simulink model "test_mdl_NI"  (R2018a)
settings: Solver=VariableStepAuto  StartTime=0.0  StopTime=10.0  RelTol=1e-3
(part 3 of 24)

== system test_mdl_NI/To_NI_HIL/MRR ==
  in : Inport
  CAN_DET_AZIMUTH_01[rad] : Subsystem
  CAN_DET_AZIMUTH_02[rad] : Subsystem
  CAN_DET_AZIMUTH_03[rad] : Subsystem
  CAN_DET_ELEVATION_01[rad] : Subsystem
  CAN_DET_ELEVATION_02[rad] : Subsystem
  CAN_DET_ELEVATION_03[rad] : Subsystem
  CAN_DET_RANGE_01[m] : Subsystem
  CAN_DET_RANGE_02[m] : Subsystem
  CAN_DET_RANGE_03[m] : Subsystem
  CAN_DET_RANGE_RATE_01[m|s] : Subsystem
  CAN_DET_RANGE_RATE_02[m|s] : Subsystem
  CAN_DET_RANGE_RATE_03[m|s] : Subsystem
  bus_creator : BusCreator  Inputs=12
  bus_selector : BusSelector  OutputSignals=CAN_DET_RANGE_01[m],CAN_DET_RANGE_RATE_01[m|s],CAN_DET_AZIMUTH_01[rad],CAN_DET_ELEVATION_01[rad],CAN_DET_RANGE_02[m],CAN_DET_RANGE_RATE_02[m|s],CAN_DET_AZIMUTH_02[rad],CAN_DET_ELEVATION_02[rad],CAN_DET_RANGE_03[m],CAN_DET_RANGE_RATE_03[m|s],CAN_DET_AZIMUTH_03[rad],CAN_DET_ELEVATION_03[rad]
  out_port : Outport
  wires:
  bus_creator/1 -> out_port/1  "MRR"
  CAN_DET_RANGE_01[m]/1(out) -> bus_creator/1  "CAN_DET_RANGE_01[m]"
  CAN_DET_RANGE_RATE_01[m|s]/1(out) -> bus_creator/2  "CAN_DET_RANGE_RATE_01[m|s]"
  CAN_DET_AZIMUTH_01[rad]/1(out) -> bus_creator/3  "CAN_DET_AZIMUTH_01[rad]"
  CAN_DET_ELEVATION_01[rad]/1(out) -> bus_creator/4  "CAN_DET_ELEVATION_01[rad]"
  CAN_DET_RANGE_02[m]/1(out) -> bus_creator/5  "CAN_DET_RANGE_02[m]"
  CAN_DET_RANGE_RATE_02[m|s]/1(out) -> bus_creator/6  "CAN_DET_RANGE_RATE_02[m|s]"
  CAN_DET_AZIMUTH_02[rad]/1(out) -> bus_creator/7  "CAN_DET_AZIMUTH_02[rad]"
  CAN_DET_ELEVATION_02[rad]/1(out) -> bus_creator/8  "CAN_DET_ELEVATION_02[rad]"
  CAN_DET_RANGE_03[m]/1(out) -> bus_creator/9  "CAN_DET_RANGE_03[m]"
  CAN_DET_RANGE_RATE_03[m|s]/1(out) -> bus_creator/10  "CAN_DET_RANGE_RATE_03[m|s]"
  CAN_DET_AZIMUTH_03[rad]/1(out) -> bus_creator/11  "CAN_DET_AZIMUTH_03[rad]"
  CAN_DET_ELEVATION_03[rad]/1(out) -> bus_creator/12  "CAN_DET_ELEVATION_03[rad]"
  bus_selector/1 -> CAN_DET_RANGE_01[m]/1(in)  "<CAN_DET_RANGE_01[m]>"
  bus_selector/2 -> CAN_DET_RANGE_RATE_01[m|s]/1(in)  "<CAN_DET_RANGE_RATE_01[m|s]>"
  bus_selector/3 -> CAN_DET_AZIMUTH_01[rad]/1(in)  "<CAN_DET_AZIMUTH_01[rad]>"
  bus_selector/4 -> CAN_DET_ELEVATION_01[rad]/1(in)  "<CAN_DET_ELEVATION_01[rad]>"
  bus_selector/5 -> CAN_DET_RANGE_02[m]/1(in)  "<CAN_DET_RANGE_02[m]>"
  bus_selector/6 -> CAN_DET_RANGE_RATE_02[m|s]/1(in)  "<CAN_DET_RANGE_RATE_02[m|s]>"
  bus_selector/7 -> CAN_DET_AZIMUTH_02[rad]/1(in)  "<CAN_DET_AZIMUTH_02[rad]>"
  bus_selector/8 -> CAN_DET_ELEVATION_02[rad]/1(in)  "<CAN_DET_ELEVATION_02[rad]>"
  bus_selector/9 -> CAN_DET_RANGE_03[m]/1(in)  "<CAN_DET_RANGE_03[m]>"
  bus_selector/10 -> CAN_DET_RANGE_RATE_03[m|s]/1(in)  "<CAN_DET_RANGE_RATE_03[m|s]>"
  bus_selector/11 -> CAN_DET_AZIMUTH_03[rad]/1(in)  "<CAN_DET_AZIMUTH_03[rad]>"
  bus_selector/12 -> CAN_DET_ELEVATION_03[rad]/1(in)  "<CAN_DET_ELEVATION_03[rad]>"
  in/1 -> bus_selector/1

== system test_mdl_NI/To_NI_HIL/SRR_L ==
  in : Inport
  FL_SOD : Subsystem
  RL_SOD : Subsystem
  bus_creator : BusCreator  Inputs=2
  bus_selector : BusSelector  OutputSignals=RL_SOD,FL_SOD
  out_port : Outport
  wires:
  bus_creator/1 -> out_port/1  "SRR_L"
  RL_SOD/1(out_port) -> bus_creator/1  "RL_SOD"
  FL_SOD/1(out_port) -> bus_creator/2  "FL_SOD"
  bus_selector/1 -> RL_SOD/1(in)  "<RL_SOD>"
  bus_selector/2 -> FL_SOD/1(in)  "<FL_SOD>"
  in/1 -> bus_selector/1

== system test_mdl_NI/To_NI_HIL/SRR_R ==
  in : Inport
  FR_SOD : Subsystem
  RR_SOD : Subsystem
  bus_creator : BusCreator  Inputs=2
  bus_selector : BusSelector  OutputSignals=RR_SOD,FR_SOD
  out_port : Outport
  wires:
  bus_creator/1 -> out_port/1  "SRR_R"
  RR_SOD/1(out_port) -> bus_creator/1  "RR_SOD"
  FR_SOD/1(out_port) -> bus_creator/2  "FR_SOD"
  bus_selector/1 -> RR_SOD/1(in)  "<RR_SOD>"
  bus_selector/2 -> FR_SOD/1(in)  "<FR_SOD>"
  in/1 -> bus_selector/1

== system test_mdl_NI/To_NI_HIL/Soft_ABS ==
  in : Inport
  ABS_BrkBst_Data : Subsystem
  Accel_Data : Subsystem
  BrakeSnData_3 : Subsystem
  BrakeSnData_4 : Subsystem
  BrakeSnData_5 : Subsystem
  BrakeSysFeatures : Subsystem
  BrakeSysFeatures_2 : Subsystem
  DesiredTorqBrk : Subsystem
  ToCarSim : Subsystem
  WheelData : Subsystem
  WheelSpeed : Subsystem
  Yaw_Data : Subsystem
  bus_creator : BusCreator  Inputs=12
  bus_selector : BusSelector  OutputSignals=WheelSpeed,WheelData,Accel_Data,Yaw_Data,BrakeSnData_3,DesiredTorqBrk,BrakeSnData_4,BrakeSysFeatures,BrakeSnData_5,ToCarSim,ABS_BrkBst_Data,BrakeSysFeatures_2
  out_port : Outport
  wires:
  bus_creator/1 -> out_port/1  "Soft_ABS"
  WheelSpeed/1(out_port) -> bus_creator/1  "WheelSpeed"
  WheelData/1(out_port) -> bus_creator/2  "WheelData"
  Accel_Data/1(out_port) -> bus_creator/3  "Accel_Data"
  Yaw_Data/1(out_port) -> bus_creator/4  "Yaw_Data"
  BrakeSnData_3/1(out_port) -> bus_creator/5  "BrakeSnData_3"
  DesiredTorqBrk/1(out_port) -> bus_creator/6  "DesiredTorqBrk"
  BrakeSnData_4/1(out_port) -> bus_creator/7  "BrakeSnData_4"
  BrakeSysFeatures/1(out_port) -> bus_creator/8  "BrakeSysFeatures"
  BrakeSnData_5/1(out_port) -> bus_creator/9  "BrakeSnData_5"
  ToCarSim/1(out_port) -> bus_creator/10  "ToCarSim"
  ABS_BrkBst_Data/1(out_port) -> bus_creator/11  "ABS_BrkBst_Data"
  BrakeSysFeatures_2/1(out_port) -> bus_creator/12  "BrakeSysFeatures_2"
  bus_selector/1 -> WheelSpeed/1(in)  "<WheelSpeed>"
  bus_selector/2 -> WheelData/1(in)  "<WheelData>"
  bus_selector/3 -> Accel_Data/1(in)  "<Accel_Data>"
  bus_selector/4 -> Yaw_Data/1(in)  "<Yaw_Data>"
  bus_selector/5 -> BrakeSnData_3/1(in)  "<BrakeSnData_3>"
  bus_selector/6 -> DesiredTorqBrk/1(in)  "<DesiredTorqBrk>"
  bus_selector/7 -> BrakeSnData_4/1(in)  "<BrakeSnData_4>"
  bus_selector/8 -> BrakeSysFeatures/1(in)  "<BrakeSysFeatures>"
  bus_selector/9 -> BrakeSnData_5/1(in)  "<BrakeSnData_5>"
  bus_selector/10 -> ToCarSim/1(in)  "<ToCarSim>"
  bus_selector/11 -> ABS_BrkBst_Data/1(in)  "<ABS_BrkBst_Data>"
  bus_selector/12 -> BrakeSysFeatures_2/1(in)  "<BrakeSysFeatures_2>"
  in/1 -> bus_selector/1

== system test_mdl_NI/To_NI_HIL/Soft_APIM ==
  in : Inport
  out : Outport
  wires:
  in/1 -> out/1

== system test_mdl_NI/To_NI_HIL/Soft_BCM ==
  in : Inport
  BodyInfo_3 : Subsystem
  Cluster_Info1 : Subsystem
  GGCC_Config_Mgmt_ID : Subsystem
  Personality_BCM2_Data : Subsystem
  bus_creator : BusCreator  Inputs=7
  bus_selector : BusSelector  OutputSignals=signal1,Cluster_Info1,BodyInfo_3,GGCC_Config_Mgmt_ID,signal5,signal6,Personality_BCM2_Data
  signal1 : Subsystem
  signal5 : Subsystem
  signal6 : Subsystem
  out_port : Outport
  wires:
  bus_creator/1 -> out_port/1  "Soft_BCM"
  signal1/1(out) -> bus_creator/1  "signal1"
  signal5/1(out) -> bus_creator/5  "signal5"
  signal6/1(out) -> bus_creator/6  "signal6"
  Cluster_Info1/1(out_port) -> bus_creator/2  "Cluster_Info1"
  BodyInfo_3/1(out_port) -> bus_creator/3  "BodyInfo_3"
  GGCC_Config_Mgmt_ID/1(out_port) -> bus_creator/4  "GGCC_Config_Mgmt_ID"
  Personality_BCM2_Data/1(out_port) -> bus_creator/7  "Personality_BCM2_Data"
  bus_selector/1 -> signal1/1(in)  "<signal1>"
  bus_selector/2 -> Cluster_Info1/1(in)  "<Cluster_Info1>"
  bus_selector/3 -> BodyInfo_3/1(in)  "<BodyInfo_3>"
  bus_selector/4 -> GGCC_Config_Mgmt_ID/1(in)  "<GGCC_Config_Mgmt_ID>"
  bus_selector/5 -> signal5/1(in)  "<signal5>"
  bus_selector/6 -> signal6/1(in)  "<signal6>"
  bus_selector/7 -> Personality_BCM2_Data/1(in)  "<Personality_BCM2_Data>"
  in/1 -> bus_selector/1

== system test_mdl_NI/To_NI_HIL/Soft_CCM ==
  in : Inport
  out : Outport
  wires:
  in/1 -> out/1

== system test_mdl_NI/To_NI_HIL/Soft_ECM ==
  in : Inport
  EngBrakeData : Subsystem
  EngVehicleSpThrottle : Subsystem
  EngVehicleSpThrottle2 : Subsystem
  bus_creator : BusCreator  Inputs=3
  bus_selector : BusSelector  OutputSignals=EngVehicleSpThrottle2,EngBrakeData,EngVehicleSpThrottle
  out_port : Outport
  wires:
  bus_creator/1 -> out_port/1  "Soft_ECM"
  EngVehicleSpThrottle2/1(out_port) -> bus_creator/1  "EngVehicleSpThrottle2"
  EngBrakeData/1(out_port) -> bus_creator/2  "EngBrakeData"
  EngVehicleSpThrottle/1(out_port) -> bus_creator/3  "EngVehicleSpThrottle"
  bus_selector/1 -> EngVehicleSpThrottle2/1(in)  "<EngVehicleSpThrottle2>"
  bus_selector/2 -> EngBrakeData/1(in)  "<EngBrakeData>"
  bus_selector/3 -> EngVehicleSpThrottle/1(in)  "<EngVehicleSpThrottle>"
  in/1 -> bus_selector/1

== system test_mdl_NI/To_NI_HIL/Soft_IPC ==
  in : Inport
  out : Outport
  wires:
  in/1 -> out/1

== system test_mdl_NI/To_NI_HIL/Soft_IPMA ==
  in : Inport
  out : Outport
  wires:
  in/1 -> out/1

== system test_mdl_NI/To_NI_HIL/Soft_MRR ==
  in : Inport
  MRR_Detection : Subsystem
  NumOfDetections : Subsystem
  bus_creator : BusCreator  Inputs=2
  bus_selector : BusSelector  OutputSignals=MRR_Detection,NumOfDetections
  out_port : Outport
  wires:
  bus_creator/1 -> out_port/1  "Soft_MRR"
  NumOfDetections/1(out) -> bus_creator/2  "NumOfDetections"
  MRR_Detection/1(out_port) -> bus_creator/1  "MRR_Detection"
  bus_selector/1 -> MRR_Detection/1(in)  "<MRR_Detection>"
  bus_selector/2 -> NumOfDetections/1(in)  "<NumOfDetections>"
  in/1 -> bus_selector/1

== system test_mdl_NI/To_NI_HIL/Soft_PCM ==
  in : Inport
  EngBrakeData : Subsystem
  EngVehicleSpThottle2 : Subsystem
  EngVehicleSpThrottle : Subsystem
  EngineClimateData : Subsystem
  EngineClutchData : Subsystem
  EngineData_7 : Subsystem
  PowertrainData_10 : Subsystem
  TorqueDataEngFlags : Subsystem
  VehicleOperatingModes : Subsystem
  bus_creator : BusCreator  Inputs=9
  bus_selector : BusSelector  OutputSignals=EngBrakeData,EngineClimateData,EngineClutchData,EngVehicleSpThrottle,EngVehicleSpThottle2,VehicleOperatingModes,EngineData_7,TorqueDataEngFlags,PowertrainData_10
  out_port : Outport
  wires:
  bus_creator/1 -> out_port/1  "Soft_PCM"
  EngBrakeData/1(out_port) -> bus_creator/1  "EngBrakeData"
  EngineClimateData/1(out_port) -> bus_creator/2  "EngineClimateData"
  EngineClutchData/1(out_port) -> bus_creator/3  "EngineClutchData"
  EngVehicleSpThrottle/1(out_port) -> bus_creator/4  "EngVehicleSpThrottle"
  EngVehicleSpThottle2/1(out_port) -> bus_creator/5  "EngVehicleSpThottle2"
  VehicleOperatingModes/1(out_port) -> bus_creator/6  "VehicleOperatingModes"
  EngineData_7/1(out_port) -> bus_creator/7  "EngineData_7"
  TorqueDataEngFlags/1(out_port) -> bus_creator/8  "TorqueDataEngFlags"
  PowertrainData_10/1(out_port) -> bus_creator/9  "PowertrainData_10"
  bus_selector/1 -> EngBrakeData/1(in)  "<EngBrakeData>"
  bus_selector/2 -> EngineClimateData/1(in)  "<EngineClimateData>"
  bus_selector/3 -> EngineClutchData/1(in)  "<EngineClutchData>"
  bus_selector/4 -> EngVehicleSpThrottle/1(in)  "<EngVehicleSpThrottle>"
  bus_selector/5 -> EngVehicleSpThottle2/1(in)  "<EngVehicleSpThottle2>"
  bus_selector/6 -> VehicleOperatingModes/1(in)  "<VehicleOperatingModes>"
  bus_selector/7 -> EngineData_7/1(in)  "<EngineData_7>"
  bus_selector/8 -> TorqueDataEngFlags/1(in)  "<TorqueDataEngFlags>"
  bus_selector/9 -> PowertrainData_10/1(in)  "<PowertrainData_10>"
  in/1 -> bus_selector/1

== system test_mdl_NI/To_NI_HIL/Soft_PSCM ==
  in : Inport
  Angle_SteeringWheel : Subsystem
  StePinCompAnEst_D_Qf : Subsystem
  StePinRelInit_An_Sns : Subsystem
  StePw_B_Rq : Subsystem
  SteWhlAngCounter : Subsystem
  WhlAngleCs : Subsystem
  bus_creator : BusCreator  Inputs=6
  bus_selector : BusSelector  OutputSignals=Angle_SteeringWheel,SteWhlAngCounter,WhlAngleCs,StePinRelInit_An_Sns,StePw_B_Rq,StePinCompAnEst_D_Qf
  out_port : Outport
  wires:
  bus_creator/1 -> out_port/1  "Soft_PSCM"
  Angle_SteeringWheel/1(out) -> bus_creator/1  "Angle_SteeringWheel"
  SteWhlAngCounter/1(out) -> bus_creator/2  "SteWhlAngCounter"
  WhlAngleCs/1(out) -> bus_creator/3  "WhlAngleCs"
  StePinRelInit_An_Sns/1(out) -> bus_creator/4  "StePinRelInit_An_Sns"
  StePw_B_Rq/1(out) -> bus_creator/5  "StePw_B_Rq"
  StePinCompAnEst_D_Qf/1(out) -> bus_creator/6  "StePinCompAnEst_D_Qf"
  bus_selector/1 -> Angle_SteeringWheel/1(in)  "<Angle_SteeringWheel>"
  bus_selector/2 -> SteWhlAngCounter/1(in)  "<SteWhlAngCounter>"
  bus_selector/3 -> WhlAngleCs/1(in)  "<WhlAngleCs>"
  bus_selector/4 -> StePinRelInit_An_Sns/1(in)  "<StePinRelInit_An_Sns>"
  bus_selector/5 -> StePw_B_Rq/1(in)  "<StePw_B_Rq>"
  bus_selector/6 -> StePinCompAnEst_D_Qf/1(in)  "<StePinCompAnEst_D_Qf>"
  in/1 -> bus_selector/1

== system test_mdl_NI/To_NI_HIL/Soft_RCM ==
  in : Inport
  Accel_Data : Subsystem
  RCMStatusMessage2 : Subsystem
  Yaw_Data : Subsystem
  bus_creator : BusCreator  Inputs=3
  bus_selector : BusSelector  OutputSignals=Accel_Data,Yaw_Data,RCMStatusMessage2
  out_port : Outport
  wires:
  bus_creator/1 -> out_port/1  "Soft_RCM"
  Accel_Data/1(out_port) -> bus_creator/1  "Accel_Data"
  Yaw_Data/1(out_port) -> bus_creator/2  "Yaw_Data"
  RCMStatusMessage2/1(out_port) -> bus_creator/3  "RCMStatusMessage2"
  bus_selector/1 -> Accel_Data/1(in)  "<Accel_Data>"
  bus_selector/2 -> Yaw_Data/1(in)  "<Yaw_Data>"
  bus_selector/3 -> RCMStatusMessage2/1(in)  "<RCMStatusMessage2>"
  in/1 -> bus_selector/1

== system test_mdl_NI/To_NI_HIL/Soft_SCCM ==
  in : Inport
  Steering_Data : Subsystem
  Steering_Wheel_Data2 : Subsystem
  bus_creator : BusCreator  Inputs=2
  bus_selector : BusSelector  OutputSignals=Steering_Data,Steering_Wheel_Data2
  out_port : Outport
  wires:
  bus_creator/1 -> out_port/1  "Soft_SCCM"
  Steering_Data/1(out_port) -> bus_creator/1  "Steering_Data"
  Steering_Wheel_Data2/1(out_port) -> bus_creator/2  "Steering_Wheel_Data2"
  bus_selector/1 -> Steering_Data/1(in)  "<Steering_Data>"
  bus_selector/2 -> Steering_Wheel_Data2/1(in)  "<Steering_Wheel_Data2>"
  in/1 -> bus_selector/1

== system test_mdl_NI/To_NI_HIL/Soft_TCM ==
  in : Inport
  TransGearData : Subsystem
  bus_creator : BusCreator  Inputs=1
  bus_selector : BusSelector  OutputSignals=TransGearData
  out_port : Outport
  wires:
  bus_creator/1 -> out_port/1  "Soft_TCM"
  TransGearData/1(out_port) -> bus_creator/1  "TransGearData"
  bus_selector/1 -> TransGearData/1(in)  "<TransGearData>"
  in/1 -> bus_selector/1

== system test_mdl_NI/CAN_Signal/ABS_ESC/ABS_AutoSar_NetworkMgt_0x596 ==
  in : Inport
  ABS_AutoSarNMControl : Subsystem
  ABS_AutoSarNMNodeId : Subsystem
  ABS_AutoSarNMReserved1 : Subsystem
  ABS_AutoSarNMReserved2 : Subsystem
  ABS_AutoSarNMReserved3 : Subsystem
  ABS_AutoSarNMReserved4 : Subsystem
  ABS_GWNMProxy : Subsystem
  ABS_GWOnBoardTester : Subsystem
  bus_creator : BusCreator  Inputs=8
  bus_selector : BusSelector  OutputSignals=ABS_AutoSarNMNodeId,ABS_AutoSarNMControl,ABS_AutoSarNMReserved1,ABS_AutoSarNMReserved2,ABS_GWOnBoardTester,ABS_GWNMProxy,ABS_AutoSarNMReserved3,ABS_AutoSarNMReserved4
  out_port : Outport
  wires:
  bus_creator/1 -> out_port/1  "ABS_AutoSar_NetworkMgt_0x596"
  ABS_AutoSarNMNodeId/1(out) -> bus_creator/1  "ABS_AutoSarNMNodeId"
  ABS_AutoSarNMControl/1(out) -> bus_creator/2  "ABS_AutoSarNMControl"
  ABS_AutoSarNMReserved1/1(out) -> bus_creator/3  "ABS_AutoSarNMReserved1"
  ABS_AutoSarNMReserved2/1(out) -> bus_creator/4  "ABS_AutoSarNMReserved2"
  ABS_GWOnBoardTester/1(out) -> bus_creator/5  "ABS_GWOnBoardTester"
  ABS_GWNMProxy/1(out) -> bus_creator/6  "ABS_GWNMProxy"
  ABS_AutoSarNMReserved3/1(out) -> bus_creator/7  "ABS_AutoSarNMReserved3"
  ABS_AutoSarNMReserved4/1(out) -> bus_creator/8  "ABS_AutoSarNMReserved4"
  bus_selector/1 -> ABS_AutoSarNMNodeId/1(in)  "<ABS_AutoSarNMNodeId>"
  bus_selector/2 -> ABS_AutoSarNMControl/1(in)  "<ABS_AutoSarNMControl>"
  bus_selector/3 -> ABS_AutoSarNMReserved1/1(in)  "<ABS_AutoSarNMReserved1>"
  bus_selector/4 -> ABS_AutoSarNMReserved2/1(in)  "<ABS_AutoSarNMReserved2>"
  bus_selector/5 -> ABS_GWOnBoardTester/1(in)  "<ABS_GWOnBoardTester>"
  bus_selector/6 -> ABS_GWNMProxy/1(in)  "<ABS_GWNMProxy>"
  bus_selector/7 -> ABS_AutoSarNMReserved3/1(in)  "<ABS_AutoSarNMReserved3>"
  bus_selector/8 -> ABS_AutoSarNMReserved4/1(in)  "<ABS_AutoSarNMReserved4>"
  in/1 -> bus_selector/1

== system test_mdl_NI/CAN_Signal/ABS_ESC/ABS_BrkBst_Data_0x4B0 ==
  in : Inport
  BrkAutoHold_D_Stat : Subsystem
  BrkBstrVac_P_Actl : Subsystem
  BrkTotTqRqDrv_No_Cnt : Subsystem
  BrkTotTqRqDrv_No_Cs : Subsystem
  BrkTot_Tq_RqDrv : Subsystem
  HsaStat_D_Dsply : Subsystem
  HsaTrnAout_Tq_Rq : Subsystem
  YawStabilityIndex : Subsystem
  bus_creator : BusCreator  Inputs=8
  bus_selector : BusSelector  OutputSignals=BrkBstrVac_P_Actl,YawStabilityIndex,HsaTrnAout_Tq_Rq,BrkTotTqRqDrv_No_Cnt,BrkAutoHold_D_Stat,BrkTot_Tq_RqDrv,HsaStat_D_Dsply,BrkTotTqRqDrv_No_Cs
  out_port : Outport
  wires:
  bus_creator/1 -> out_port/1  "ABS_BrkBst_Data_0x4B0"
  BrkBstrVac_P_Actl/1(out) -> bus_creator/1  "BrkBstrVac_P_Actl"
  YawStabilityIndex/1(out) -> bus_creator/2  "YawStabilityIndex"
  HsaTrnAout_Tq_Rq/1(out) -> bus_creator/3  "HsaTrnAout_Tq_Rq"
  BrkTotTqRqDrv_No_Cnt/1(out) -> bus_creator/4  "BrkTotTqRqDrv_No_Cnt"
  BrkAutoHold_D_Stat/1(out) -> bus_creator/5  "BrkAutoHold_D_Stat"
  BrkTot_Tq_RqDrv/1(out) -> bus_creator/6  "BrkTot_Tq_RqDrv"
  HsaStat_D_Dsply/1(out) -> bus_creator/7  "HsaStat_D_Dsply"
  BrkTotTqRqDrv_No_Cs/1(out) -> bus_creator/8  "BrkTotTqRqDrv_No_Cs"
  bus_selector/1 -> BrkBstrVac_P_Actl/1(in)  "<BrkBstrVac_P_Actl>"
  bus_selector/2 -> YawStabilityIndex/1(in)  "<YawStabilityIndex>"
  bus_selector/3 -> HsaTrnAout_Tq_Rq/1(in)  "<HsaTrnAout_Tq_Rq>"
  bus_selector/4 -> BrkTotTqRqDrv_No_Cnt/1(in)  "<BrkTotTqRqDrv_No_Cnt>"
  bus_selector/5 -> BrkAutoHold_D_Stat/1(in)  "<BrkAutoHold_D_Stat>"
  bus_selector/6 -> BrkTot_Tq_RqDrv/1(in)  "<BrkTot_Tq_RqDrv>"
  bus_selector/7 -> HsaStat_D_Dsply/1(in)  "<HsaStat_D_Dsply>"
  bus_selector/8 -> BrkTotTqRqDrv_No_Cs/1(in)  "<BrkTotTqRqDrv_No_Cs>"
  in/1 -> bus_selector/1

== system test_mdl_NI/CAN_Signal/ABS_ESC/ABS_Rapid_Data_Response_1_0x6B0 ==
  in : Inport
  UUDTABSResponse1 : Subsystem
  bus_creator : BusCreator  Inputs=1
  bus_selector : BusSelector  OutputSignals=UUDTABSResponse1
  out_port : Outport
  wires:
  bus_creator/1 -> out_port/1  "ABS_Rapid_Data_Response_1_0x6B0"
  UUDTABSResponse1/1(out) -> bus_creator/1  "UUDTABSResponse1"
  bus_selector/1 -> UUDTABSResponse1/1(in)  "<UUDTABSResponse1>"
  in/1 -> bus_selector/1

== system test_mdl_NI/CAN_Signal/ABS_ESC/ABS_Rapid_Data_Response_2_0x6B1 ==
  in : Inport
  UUDTABSResponse2 : Subsystem
  bus_creator : BusCreator  Inputs=1
  bus_selector : BusSelector  OutputSignals=UUDTABSResponse2
  out_port : Outport
  wires:
  bus_creator/1 -> out_port/1  "ABS_Rapid_Data_Response_2_0x6B1"
  UUDTABSResponse2/1(out) -> bus_creator/1  "UUDTABSResponse2"
  bus_selector/1 -> UUDTABSResponse2/1(in)  "<UUDTABSResponse2>"
  in/1 -> bus_selector/1

== system test_mdl_NI/CAN_Signal/ABS_ESC/ActiveFronSteering_Req_0x88 ==
  in : Inport
  SteWhlBrkAnRq_No_Cnt : Subsystem
  SteWhlBrkAnRq_No_Cs : Subsystem
  SteWhlBrkOffst_An_Rq : Subsystem
  bus_creator : BusCreator  Inputs=3
  bus_selector : BusSelector  OutputSignals=SteWhlBrkOffst_An_Rq,SteWhlBrkAnRq_No_Cs,SteWhlBrkAnRq_No_Cnt
  out_port : Outport
  wires:
  bus_creator/1 -> out_port/1  "ActiveFronSteering_Req_0x88"
  SteWhlBrkOffst_An_Rq/1(out) -> bus_creator/1  "SteWhlBrkOffst_An_Rq"
  SteWhlBrkAnRq_No_Cs/1(out) -> bus_creator/2  "SteWhlBrkAnRq_No_Cs"
  SteWhlBrkAnRq_No_Cnt/1(out) -> bus_creator/3  "SteWhlBrkAnRq_No_Cnt"
  bus_selector/1 -> SteWhlBrkOffst_An_Rq/1(in)  "<SteWhlBrkOffst_An_Rq>"
  bus_selector/2 -> SteWhlBrkAnRq_No_Cs/1(in)  "<SteWhlBrkAnRq_No_Cs>"
  bus_selector/3 -> SteWhlBrkAnRq_No_Cnt/1(in)  "<SteWhlBrkAnRq_No_Cnt>"
  in/1 -> bus_selector/1

== system test_mdl_NI/CAN_Signal/ABS_ESC/BrakeSnData_3_0x77 ==
  in : Inport
  VehLatComp_A_Actl : Subsystem
  VehLongComp_A_Actl : Subsystem
  VehOverGnd_V_Est : Subsystem
  VehTrvlDir_D_Stat : Subsystem
  VehYawComp_W_Actl : Subsystem
  bus_creator : BusCreator  Inputs=5
  bus_selector : BusSelector  OutputSignals=VehOverGnd_V_Est,VehTrvlDir_D_Stat,VehYawComp_W_Actl,VehLatComp_A_Actl,VehLongComp_A_Actl
  out_port : Outport
  wires:
  bus_creator/1 -> out_port/1  "BrakeSnData_3_0x77"
  VehOverGnd_V_Est/1(out) -> bus_creator/1  "VehOverGnd_V_Est"
  VehTrvlDir_D_Stat/1(out) -> bus_creator/2  "VehTrvlDir_D_Stat"
  VehYawComp_W_Actl/1(out) -> bus_creator/3  "VehYawComp_W_Actl"
  VehLatComp_A_Actl/1(out) -> bus_creator/4  "VehLatComp_A_Actl"
  VehLongComp_A_Actl/1(out) -> bus_creator/5  "VehLongComp_A_Actl"
  bus_selector/1 -> VehOverGnd_V_Est/1(in)  "<VehOverGnd_V_Est>"
  bus_selector/2 -> VehTrvlDir_D_Stat/1(in)  "<VehTrvlDir_D_Stat>"
  bus_selector/3 -> VehYawComp_W_Actl/1(in)  "<VehYawComp_W_Actl>"
  bus_selector/4 -> VehLatComp_A_Actl/1(in)  "<VehLatComp_A_Actl>"
  bus_selector/5 -> VehLongComp_A_Actl/1(in)  "<VehLongComp_A_Actl>"
  in/1 -> bus_selector/1

== system test_mdl_NI/CAN_Signal/ABS_ESC/BrakeSnData_4_0x7D ==
  in : Inport
  BrkTotTqRqArb_No_Cnt : Subsystem
  BrkTotTqRqArb_No_Cs : Subsystem
  BrkTot_Tq_Actl : Subsystem
  BrkTot_Tq_RqArb : Subsystem
  HsaStat_D_Actl : Subsystem
  VehRolComp_W_Actl : Subsystem
  VehVertComp_A_Actl : Subsystem
  bus_creator : BusCreator  Inputs=7
  bus_selector : BusSelector  OutputSignals=HsaStat_D_Actl,BrkTot_Tq_RqArb,BrkTotTqRqArb_No_Cs,BrkTotTqRqArb_No_Cnt,BrkTot_Tq_Actl,VehVertComp_A_Actl,VehRolComp_W_Actl
  out_port : Outport
  wires:
  bus_creator/1 -> out_port/1  "BrakeSnData_4_0x7D"
  HsaStat_D_Actl/1(out) -> bus_creator/1  "HsaStat_D_Actl"
  BrkTot_Tq_RqArb/1(out) -> bus_creator/2  "BrkTot_Tq_RqArb"
  BrkTotTqRqArb_No_Cs/1(out) -> bus_creator/3  "BrkTotTqRqArb_No_Cs"
  BrkTotTqRqArb_No_Cnt/1(out) -> bus_creator/4  "BrkTotTqRqArb_No_Cnt"
  BrkTot_Tq_Actl/1(out) -> bus_creator/5  "BrkTot_Tq_Actl"
  VehVertComp_A_Actl/1(out) -> bus_creator/6  "VehVertComp_A_Actl"
  VehRolComp_W_Actl/1(out) -> bus_creator/7  "VehRolComp_W_Actl"
  bus_selector/1 -> HsaStat_D_Actl/1(in)  "<HsaStat_D_Actl>"
  bus_selector/2 -> BrkTot_Tq_RqArb/1(in)  "<BrkTot_Tq_RqArb>"
  bus_selector/3 -> BrkTotTqRqArb_No_Cs/1(in)  "<BrkTotTqRqArb_No_Cs>"
  bus_selector/4 -> BrkTotTqRqArb_No_Cnt/1(in)  "<BrkTotTqRqArb_No_Cnt>"
  bus_selector/5 -> BrkTot_Tq_Actl/1(in)  "<BrkTot_Tq_Actl>"
  bus_selector/6 -> VehVertComp_A_Actl/1(in)  "<VehVertComp_A_Actl>"
  bus_selector/7 -> VehRolComp_W_Actl/1(in)  "<VehRolComp_W_Actl>"
  in/1 -> bus_selector/1

== system test_mdl_NI/CAN_Signal/ABS_ESC/BrakeSnData_5_0x76 ==
  in : Inport
  AwdLck_Tq_RqMn : Subsystem
  AwdLck_Tq_RqMx : Subsystem
  BrkCtrFnd_B_Stat : Subsystem
  DrvSte_D_Stat : Subsystem
  DrvSte_Tq_Rq : Subsystem
  EmgcyBrkLamp_D_Rq : Subsystem
  SteWhlCompAnEst_D_Qf : Subsystem
  SteWhlComp_An_Est : Subsystem
  StopLamp_B_RqBrk : Subsystem
  bus_creator : BusCreator  Inputs=9
  bus_selector : BusSelector  OutputSignals=StopLamp_B_RqBrk,SteWhlComp_An_Est,SteWhlCompAnEst_D_Qf,EmgcyBrkLamp_D_Rq,DrvSte_D_Stat,DrvSte_Tq_Rq,BrkCtrFnd_B_Stat,AwdLck_Tq_RqMx,AwdLck_Tq_RqMn
  out_port : Outport
  wires:
  bus_creator/1 -> out_port/1  "BrakeSnData_5_0x76"
  StopLamp_B_RqBrk/1(out) -> bus_creator/1  "StopLamp_B_RqBrk"
  SteWhlComp_An_Est/1(out) -> bus_creator/2  "SteWhlComp_An_Est"
  SteWhlCompAnEst_D_Qf/1(out) -> bus_creator/3  "SteWhlCompAnEst_D_Qf"
  EmgcyBrkLamp_D_Rq/1(out) -> bus_creator/4  "EmgcyBrkLamp_D_Rq"
  DrvSte_D_Stat/1(out) -> bus_creator/5  "DrvSte_D_Stat"
  DrvSte_Tq_Rq/1(out) -> bus_creator/6  "DrvSte_Tq_Rq"
  BrkCtrFnd_B_Stat/1(out) -> bus_creator/7  "BrkCtrFnd_B_Stat"
  AwdLck_Tq_RqMx/1(out) -> bus_creator/8  "AwdLck_Tq_RqMx"
  AwdLck_Tq_RqMn/1(out) -> bus_creator/9  "AwdLck_Tq_RqMn"
  bus_selector/1 -> StopLamp_B_RqBrk/1(in)  "<StopLamp_B_RqBrk>"
  bus_selector/2 -> SteWhlComp_An_Est/1(in)  "<SteWhlComp_An_Est>"
  bus_selector/3 -> SteWhlCompAnEst_D_Qf/1(in)  "<SteWhlCompAnEst_D_Qf>"
  bus_selector/4 -> EmgcyBrkLamp_D_Rq/1(in)  "<EmgcyBrkLamp_D_Rq>"
  bus_selector/5 -> DrvSte_D_Stat/1(in)  "<DrvSte_D_Stat>"
  bus_selector/6 -> DrvSte_Tq_Rq/1(in)  "<DrvSte_Tq_Rq>"
  bus_selector/7 -> BrkCtrFnd_B_Stat/1(in)  "<BrkCtrFnd_B_Stat>"
  bus_selector/8 -> AwdLck_Tq_RqMx/1(in)  "<AwdLck_Tq_RqMx>"
  bus_selector/9 -> AwdLck_Tq_RqMn/1(in)  "<AwdLck_Tq_RqMn>"
  in/1 -> bus_selector/1

== system test_mdl_NI/CAN_Signal/ABS_ESC/BrakeSnData_6_0x414 ==
  in : Inport
  StePinOffst_An_Est : Subsystem
  StePinOffst_D_Stat : Subsystem
  StePinOffst_No_Cnt : Subsystem
  StePinOffst_No_Cs : Subsystem
  bus_creator : BusCreator  Inputs=4
  bus_selector : BusSelector  OutputSignals=StePinOffst_An_Est,StePinOffst_D_Stat,StePinOffst_No_Cnt,StePinOffst_No_Cs
  out_port : Outport
  wires:
  bus_creator/1 -> out_port/1  "BrakeSnData_6_0x414"
  StePinOffst_An_Est/1(out) -> bus_creator/1  "StePinOffst_An_Est"
  StePinOffst_D_Stat/1(out) -> bus_creator/2  "StePinOffst_D_Stat"
  StePinOffst_No_Cnt/1(out) -> bus_creator/3  "StePinOffst_No_Cnt"
  StePinOffst_No_Cs/1(out) -> bus_creator/4  "StePinOffst_No_Cs"
  bus_selector/1 -> StePinOffst_An_Est/1(in)  "<StePinOffst_An_Est>"
  bus_selector/2 -> StePinOffst_D_Stat/1(in)  "<StePinOffst_D_Stat>"
  bus_selector/3 -> StePinOffst_No_Cnt/1(in)  "<StePinOffst_No_Cnt>"
  bus_selector/4 -> StePinOffst_No_Cs/1(in)  "<StePinOffst_No_Cs>"
  in/1 -> bus_selector/1

== system test_mdl_NI/CAN_Signal/ABS_ESC/BrakeSysFeatures_0x415 ==
  in : Inport
  BrkFluidLvl_D_Stat : Subsystem
  LsmcBrkDecel_D_Stat : Subsystem
  VehStab_D_Stat : Subsystem
  VehVActlBrk_D_Qf : Subsystem
  VehVActlBrk_No_Cnt : Subsystem
  VehVActlBrk_No_Cs : Subsystem
  VehYawLin_W_Rq : Subsystem
  VehYawNonLin_W_Rq : Subsystem
  Veh_V_ActlBrk : Subsystem
  bus_creator : BusCreator  Inputs=9
  bus_selector : BusSelector  OutputSignals=Veh_V_ActlBrk,VehVActlBrk_D_Qf,VehVActlBrk_No_Cnt,BrkFluidLvl_D_Stat,VehVActlBrk_No_Cs,LsmcBrkDecel_D_Stat,VehYawLin_W_Rq,VehStab_D_Stat,VehYawNonLin_W_Rq
  out_port : Outport
  wires:
  bus_creator/1 -> out_port/1  "BrakeSysFeatures_0x415"
  Veh_V_ActlBrk/1(out) -> bus_creator/1  "Veh_V_ActlBrk"
  VehVActlBrk_D_Qf/1(out) -> bus_creator/2  "VehVActlBrk_D_Qf"
  VehVActlBrk_No_Cnt/1(out) -> bus_creator/3  "VehVActlBrk_No_Cnt"
  BrkFluidLvl_D_Stat/1(out) -> bus_creator/4  "BrkFluidLvl_D_Stat"
  VehVActlBrk_No_Cs/1(out) -> bus_creator/5  "VehVActlBrk_No_Cs"
  LsmcBrkDecel_D_Stat/1(out) -> bus_creator/6  "LsmcBrkDecel_D_Stat"
  VehYawLin_W_Rq/1(out) -> bus_creator/7  "VehYawLin_W_Rq"
  VehStab_D_Stat/1(out) -> bus_creator/8  "VehStab_D_Stat"
  VehYawNonLin_W_Rq/1(out) -> bus_creator/9  "VehYawNonLin_W_Rq"
  bus_selector/1 -> Veh_V_ActlBrk/1(in)  "<Veh_V_ActlBrk>"
  bus_selector/2 -> VehVActlBrk_D_Qf/1(in)  "<VehVActlBrk_D_Qf>"
  bus_selector/3 -> VehVActlBrk_No_Cnt/1(in)  "<VehVActlBrk_No_Cnt>"
  bus_selector/4 -> BrkFluidLvl_D_Stat/1(in)  "<BrkFluidLvl_D_Stat>"
  bus_selector/5 -> VehVActlBrk_No_Cs/1(in)  "<VehVActlBrk_No_Cs>"
  bus_selector/6 -> LsmcBrkDecel_D_Stat/1(in)  "<LsmcBrkDecel_D_Stat>"
  bus_selector/7 -> VehYawLin_W_Rq/1(in)  "<VehYawLin_W_Rq>"
  bus_selector/8 -> VehStab_D_Stat/1(in)  "<VehStab_D_Stat>"
  bus_selector/9 -> VehYawNonLin_W_Rq/1(in)  "<VehYawNonLin_W_Rq>"
  in/1 -> bus_selector/1

== system test_mdl_NI/CAN_Signal/ABS_ESC/BrakeSysFeatures_2_0x416 ==
  in : Inport
  Abs_B_Falt : Subsystem
  BpedMove_D_Actl : Subsystem
  BpedMove_No_Cnt : Subsystem
  BrkBstrVac_B_Rq : Subsystem
  BrkLamp_B_Rq : Subsystem
  ChimeBrk_B_Rq : Subsystem
  DrvAntiLckLamp_D_Rq : Subsystem
  DrvHdcLampInfo_D_Rq : Subsystem
  DrvHdcMsg_D_Rq : Subsystem
  DrvHdcWarnInfo_D_Rq : Subsystem
  DrvSlipCtlLamp_D_Rq : Subsystem
  DrvSlipCtlMde_D_Ind : Subsystem
  HILL_DESC_MC : Subsystem
  HdcMde_D_Actl : Subsystem
  HsaMde_D_Mem : Subsystem
  RearDiffElckrOpen_B_Rq : Subsystem
  RearDiffLck_Tq2_RqMx : Subsystem
  StabCtlBrk_B_Avail : Subsystem
  TCMode : Subsystem
  TRLR_SWAY_CONFIG_STAT : Subsystem
  TRLR_SWAY_EVNT_IN_PROG : Subsystem
  bus_creator : BusCreator  Inputs=21
  bus_selector : BusSelector  OutputSignals=BpedMove_D_Actl,Abs_B_Falt,StabCtlBrk_B_Avail,BpedMove_No_Cnt,TCMode,ChimeBrk_B_Rq,BrkLamp_B_Rq,DrvHdcLampInfo_D_Rq,DrvHdcMsg_D_Rq,HdcMde_D_Actl,BrkBstrVac_B_Rq,TRLR_SWAY_CONFIG_STAT,TRLR_SWAY_EVNT_IN_PROG,DrvHdcWarnInfo_D_Rq,HsaMde_D_Mem,HILL_DESC_MC,DrvSlipCtlMde_D_Ind,DrvSlipCtlLamp_D_Rq,RearDiffElckrOpen_B_Rq,DrvAntiLckLamp_D_Rq,RearDiffLck_Tq2_RqMx
  out_port : Outport
  wires:
  bus_creator/1 -> out_port/1  "BrakeSysFeatures_2_0x416"
  BpedMove_D_Actl/1(out) -> bus_creator/1  "BpedMove_D_Actl"
  Abs_B_Falt/1(out) -> bus_creator/2  "Abs_B_Falt"
  StabCtlBrk_B_Avail/1(out) -> bus_creator/3  "StabCtlBrk_B_Avail"
  BpedMove_No_Cnt/1(out) -> bus_creator/4  "BpedMove_No_Cnt"
  TCMode/1(out) -> bus_creator/5  "TCMode"
  ChimeBrk_B_Rq/1(out) -> bus_creator/6  "ChimeBrk_B_Rq"
  BrkLamp_B_Rq/1(out) -> bus_creator/7  "BrkLamp_B_Rq"
  DrvHdcLampInfo_D_Rq/1(out) -> bus_creator/8  "DrvHdcLampInfo_D_Rq"
  DrvHdcMsg_D_Rq/1(out) -> bus_creator/9  "DrvHdcMsg_D_Rq"
  HdcMde_D_Actl/1(out) -> bus_creator/10  "HdcMde_D_Actl"
  BrkBstrVac_B_Rq/1(out) -> bus_creator/11  "BrkBstrVac_B_Rq"
  TRLR_SWAY_CONFIG_STAT/1(out) -> bus_creator/12  "TRLR_SWAY_CONFIG_STAT"
  TRLR_SWAY_EVNT_IN_PROG/1(out) -> bus_creator/13  "TRLR_SWAY_EVNT_IN_PROG"
  DrvHdcWarnInfo_D_Rq/1(out) -> bus_creator/14  "DrvHdcWarnInfo_D_Rq"
  HsaMde_D_Mem/1(out) -> bus_creator/15  "HsaMde_D_Mem"
  HILL_DESC_MC/1(out) -> bus_creator/16  "HILL_DESC_MC"
  DrvSlipCtlMde_D_Ind/1(out) -> bus_creator/17  "DrvSlipCtlMde_D_Ind"
  DrvSlipCtlLamp_D_Rq/1(out) -> bus_creator/18  "DrvSlipCtlLamp_D_Rq"
  RearDiffElckrOpen_B_Rq/1(out) -> bus_creator/19  "RearDiffElckrOpen_B_Rq"
  DrvAntiLckLamp_D_Rq/1(out) -> bus_creator/20  "DrvAntiLckLamp_D_Rq"
  RearDiffLck_Tq2_RqMx/1(out) -> bus_creator/21  "RearDiffLck_Tq2_RqMx"
  bus_selector/1 -> BpedMove_D_Actl/1(in)  "<BpedMove_D_Actl>"
  bus_selector/2 -> Abs_B_Falt/1(in)  "<Abs_B_Falt>"
  bus_selector/3 -> StabCtlBrk_B_Avail/1(in)  "<StabCtlBrk_B_Avail>"
  bus_selector/4 -> BpedMove_No_Cnt/1(in)  "<BpedMove_No_Cnt>"
  bus_selector/5 -> TCMode/1(in)  "<TCMode>"
  bus_selector/6 -> ChimeBrk_B_Rq/1(in)  "<ChimeBrk_B_Rq>"
  bus_selector/7 -> BrkLamp_B_Rq/1(in)  "<BrkLamp_B_Rq>"
  bus_selector/8 -> DrvHdcLampInfo_D_Rq/1(in)  "<DrvHdcLampInfo_D_Rq>"
  bus_selector/9 -> DrvHdcMsg_D_Rq/1(in)  "<DrvHdcMsg_D_Rq>"
  bus_selector/10 -> HdcMde_D_Actl/1(in)  "<HdcMde_D_Actl>"
  bus_selector/11 -> BrkBstrVac_B_Rq/1(in)  "<BrkBstrVac_B_Rq>"
  bus_selector/12 -> TRLR_SWAY_CONFIG_STAT/1(in)  "<TRLR_SWAY_CONFIG_STAT>"
  bus_selector/13 -> TRLR_SWAY_EVNT_IN_PROG/1(in)  "<TRLR_SWAY_EVNT_IN_PROG>"
  bus_selector/14 -> DrvHdcWarnInfo_D_Rq/1(in)  "<DrvHdcWarnInfo_D_Rq>"
  bus_selector/15 -> HsaMde_D_Mem/1(in)  "<HsaMde_D_Mem>"
  bus_selector/16 -> HILL_DESC_MC/1(in)  "<HILL_DESC_MC>"
  bus_selector/17 -> DrvSlipCtlMde_D_Ind/1(in)  "<DrvSlipCtlMde_D_Ind>"
  bus_selector/18 -> DrvSlipCtlLamp_D_Rq/1(in)  "<DrvSlipCtlLamp_D_Rq>"
  bus_selector/19 -> RearDiffElckrOpen_B_Rq/1(in)  "<RearDiffElckrOpen_B_Rq>"
  bus_selector/20 -> DrvAntiLckLamp_D_Rq/1(in)  "<DrvAntiLckLamp_D_Rq>"
  bus_selector/21 -> RearDiffLck_Tq2_RqMx/1(in)  "<RearDiffLck_Tq2_RqMx>"
  in/1 -> bus_selector/1

== system test_mdl_NI/CAN_Signal/ABS_ESC/BrakeSysFeatures_3_0x41E ==
  in : Inport
  ApaBrk_D_Stat : Subsystem
  AutoHoldMde_D_Ind : Subsystem
  AutoHoldMsgTxt_D_Rq : Subsystem
  AutoHoldSwMde_B_Ind : Subsystem
  BrkBstrVac_D_Stat : Subsystem
  BrkMdeInhbt_B_RqDsply : Subsystem
  CtaBrk_D_Stat : Subsystem
  DrvSlipCtlMdeMsg_D_Rq : Subsystem
  DrvSlipCtlOffLamp_D_Rq : Subsystem
  RbaBrk_D_Stat : Subsystem
  SelDrvMdeAwd_D_Rq : Subsystem
  SelDrvMdeChassis2_D_Rq : Subsystem
  SelDrvMdeChassis_D_Rq : Subsystem
  TrailCtlMsgTxt_D_Rq : Subsystem
  TrailCtl_D_Stat : Subsystem
  bus_creator : BusCreator  Inputs=15
  bus_selector : BusSelector  OutputSignals=AutoHoldMsgTxt_D_Rq,AutoHoldSwMde_B_Ind,AutoHoldMde_D_Ind,DrvSlipCtlMdeMsg_D_Rq,BrkMdeInhbt_B_RqDsply,DrvSlipCtlOffLamp_D_Rq,BrkBstrVac_D_Stat,SelDrvMdeAwd_D_Rq,SelDrvMdeChassis_D_Rq,ApaBrk_D_Stat,CtaBrk_D_Stat,SelDrvMdeChassis2_D_Rq,TrailCtl_D_Stat,TrailCtlMsgTxt_D_Rq,RbaBrk_D_Stat
  out_port : Outport
  wires:
  bus_creator/1 -> out_port/1  "BrakeSysFeatures_3_0x41E"
  AutoHoldMsgTxt_D_Rq/1(out) -> bus_creator/1  "AutoHoldMsgTxt_D_Rq"
  AutoHoldSwMde_B_Ind/1(out) -> bus_creator/2  "AutoHoldSwMde_B_Ind"
  AutoHoldMde_D_Ind/1(out) -> bus_creator/3  "AutoHoldMde_D_Ind"
  DrvSlipCtlMdeMsg_D_Rq/1(out) -> bus_creator/4  "DrvSlipCtlMdeMsg_D_Rq"
  BrkMdeInhbt_B_RqDsply/1(out) -> bus_creator/5  "BrkMdeInhbt_B_RqDsply"
  DrvSlipCtlOffLamp_D_Rq/1(out) -> bus_creator/6  "DrvSlipCtlOffLamp_D_Rq"
  BrkBstrVac_D_Stat/1(out) -> bus_creator/7  "BrkBstrVac_D_Stat"
  SelDrvMdeAwd_D_Rq/1(out) -> bus_creator/8  "SelDrvMdeAwd_D_Rq"
  SelDrvMdeChassis_D_Rq/1(out) -> bus_creator/9  "SelDrvMdeChassis_D_Rq"
  ApaBrk_D_Stat/1(out) -> bus_creator/10  "ApaBrk_D_Stat"
  CtaBrk_D_Stat/1(out) -> bus_creator/11  "CtaBrk_D_Stat"
  SelDrvMdeChassis2_D_Rq/1(out) -> bus_creator/12  "SelDrvMdeChassis2_D_Rq"
  TrailCtl_D_Stat/1(out) -> bus_creator/13  "TrailCtl_D_Stat"
  TrailCtlMsgTxt_D_Rq/1(out) -> bus_creator/14  "TrailCtlMsgTxt_D_Rq"
  RbaBrk_D_Stat/1(out) -> bus_creator/15  "RbaBrk_D_Stat"
  bus_selector/1 -> AutoHoldMsgTxt_D_Rq/1(in)  "<AutoHoldMsgTxt_D_Rq>"
  bus_selector/2 -> AutoHoldSwMde_B_Ind/1(in)  "<AutoHoldSwMde_B_Ind>"
  bus_selector/3 -> AutoHoldMde_D_Ind/1(in)  "<AutoHoldMde_D_Ind>"
  bus_selector/4 -> DrvSlipCtlMdeMsg_D_Rq/1(in)  "<DrvSlipCtlMdeMsg_D_Rq>"
  bus_selector/5 -> BrkMdeInhbt_B_RqDsply/1(in)  "<BrkMdeInhbt_B_RqDsply>"
  bus_selector/6 -> DrvSlipCtlOffLamp_D_Rq/1(in)  "<DrvSlipCtlOffLamp_D_Rq>"
  bus_selector/7 -> BrkBstrVac_D_Stat/1(in)  "<BrkBstrVac_D_Stat>"
  bus_selector/8 -> SelDrvMdeAwd_D_Rq/1(in)  "<SelDrvMdeAwd_D_Rq>"
  bus_selector/9 -> SelDrvMdeChassis_D_Rq/1(in)  "<SelDrvMdeChassis_D_Rq>"
  bus_selector/10 -> ApaBrk_D_Stat/1(in)  "<ApaBrk_D_Stat>"
  bus_selector/11 -> CtaBrk_D_Stat/1(in)  "<CtaBrk_D_Stat>"
  bus_selector/12 -> SelDrvMdeChassis2_D_Rq/1(in)  "<SelDrvMdeChassis2_D_Rq>"
  bus_selector/13 -> TrailCtl_D_Stat/1(in)  "<TrailCtl_D_Stat>"
  bus_selector/14 -> TrailCtlMsgTxt_D_Rq/1(in)  "<TrailCtlMsgTxt_D_Rq>"
  bus_selector/15 -> RbaBrk_D_Stat/1(in)  "<RbaBrk_D_Stat>"
  in/1 -> bus_selector/1

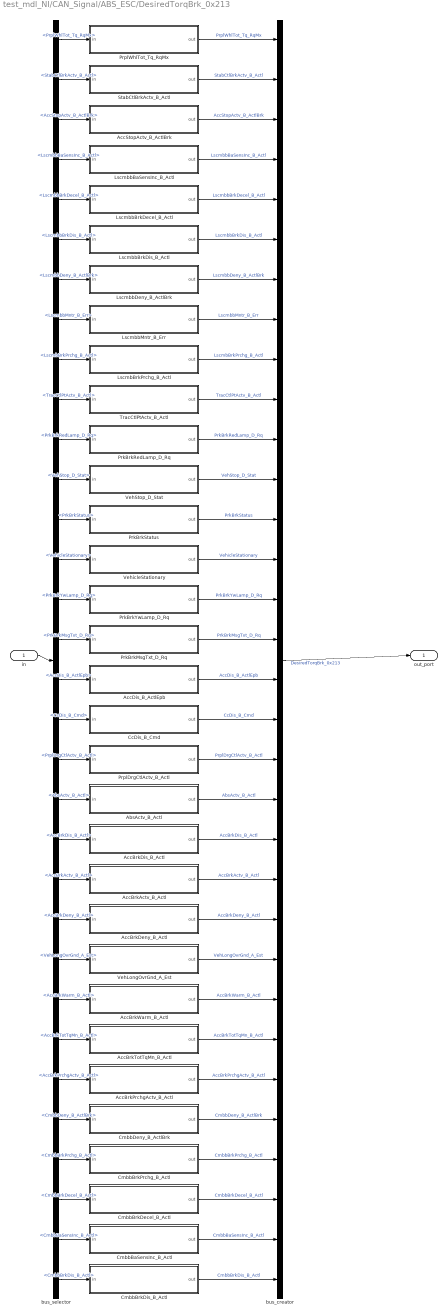
== system test_mdl_NI/CAN_Signal/ABS_ESC/DesiredTorqBrk_0x213 ==
  in : Inport
  AbsActv_B_Actl : Subsystem
  AccBrkActv_B_Actl : Subsystem
  AccBrkDeny_B_Actl : Subsystem
  AccBrkDis_B_Actl : Subsystem
  AccBrkPrchgActv_B_Actl : Subsystem
  AccBrkTotTqMn_B_Actl : Subsystem
  AccBrkWarm_B_Actl : Subsystem
  AccDis_B_ActlEpb : Subsystem
  AccStopActv_B_ActlBrk : Subsystem
  CcDis_B_Cmd : Subsystem
  CmbbBaSensInc_B_Actl : Subsystem
  CmbbBrkDecel_B_Actl : Subsystem
  CmbbBrkDis_B_Actl : Subsystem
  CmbbBrkPrchg_B_Actl : Subsystem
  CmbbDeny_B_ActlBrk : Subsystem
  LscmbBrkPrchg_B_Actl : Subsystem
  LscmbbBaSensInc_B_Actl : Subsystem
  LscmbbBrkDecel_B_Actl : Subsystem
  LscmbbBrkDis_B_Actl : Subsystem
  LscmbbDeny_B_ActlBrk : Subsystem
  LscmbbMntr_B_Err : Subsystem
  PrkBrkMsgTxt_D_Rq : Subsystem
  PrkBrkRedLamp_D_Rq : Subsystem
  PrkBrkStatus : Subsystem
  PrkBrkYwLamp_D_Rq : Subsystem
  PrplDrgCtlActv_B_Actl : Subsystem
  PrplWhlTot_Tq_RqMx : Subsystem
  StabCtlBrkActv_B_Actl : Subsystem
  TracCtlPtActv_B_Actl : Subsystem
  VehLongOvrGnd_A_Est : Subsystem
  VehStop_D_Stat : Subsystem
  VehicleStationary : Subsystem
  bus_creator : BusCreator  Inputs=32
  bus_selector : BusSelector  OutputSignals=PrplWhlTot_Tq_RqMx,StabCtlBrkActv_B_Actl,AccStopActv_B_ActlBrk,LscmbbBaSensInc_B_Actl,LscmbbBrkDecel_B_Actl,LscmbbBrkDis_B_Actl,LscmbbDeny_B_ActlBrk,LscmbbMntr_B_Err,LscmbBrkPrchg_B_Actl,TracCtlPtActv_B_Actl,PrkBrkRedLamp_D_Rq,VehStop_D_Stat,PrkBrkStatus,VehicleStationary,PrkBrkYwLamp_D_Rq,PrkBrkMsgTxt_D_Rq,AccDis_B_ActlEpb,CcDis_B_Cmd,PrplDrgCtlActv_B_Actl,AbsActv_B_Actl,AccBrkDis_B_Actl,AccBrkActv_B_Actl,AccBrkDeny_B_Actl,VehLongOvrGnd_A_Est,AccBrkWarm_B_Actl,AccBrkTotTqMn_B_Actl,AccBrkPrchgActv_B_Actl,CmbbDeny_B_ActlBrk,CmbbBrkPrchg_B_Actl,CmbbBrkDecel_B_Actl,CmbbBaSensInc_B_Actl,CmbbBrkDis_B_Actl
  out_port : Outport
  wires:
  bus_creator/1 -> out_port/1  "DesiredTorqBrk_0x213"
  PrplWhlTot_Tq_RqMx/1(out) -> bus_creator/1  "PrplWhlTot_Tq_RqMx"
  StabCtlBrkActv_B_Actl/1(out) -> bus_creator/2  "StabCtlBrkActv_B_Actl"
  AccStopActv_B_ActlBrk/1(out) -> bus_creator/3  "AccStopActv_B_ActlBrk"
  LscmbbBaSensInc_B_Actl/1(out) -> bus_creator/4  "LscmbbBaSensInc_B_Actl"
  LscmbbBrkDecel_B_Actl/1(out) -> bus_creator/5  "LscmbbBrkDecel_B_Actl"
  LscmbbBrkDis_B_Actl/1(out) -> bus_creator/6  "LscmbbBrkDis_B_Actl"
  LscmbbDeny_B_ActlBrk/1(out) -> bus_creator/7  "LscmbbDeny_B_ActlBrk"
  LscmbbMntr_B_Err/1(out) -> bus_creator/8  "LscmbbMntr_B_Err"
  LscmbBrkPrchg_B_Actl/1(out) -> bus_creator/9  "LscmbBrkPrchg_B_Actl"
  TracCtlPtActv_B_Actl/1(out) -> bus_creator/10  "TracCtlPtActv_B_Actl"
  PrkBrkRedLamp_D_Rq/1(out) -> bus_creator/11  "PrkBrkRedLamp_D_Rq"
  VehStop_D_Stat/1(out) -> bus_creator/12  "VehStop_D_Stat"
  PrkBrkStatus/1(out) -> bus_creator/13  "PrkBrkStatus"
  VehicleStationary/1(out) -> bus_creator/14  "VehicleStationary"
  PrkBrkYwLamp_D_Rq/1(out) -> bus_creator/15  "PrkBrkYwLamp_D_Rq"
  PrkBrkMsgTxt_D_Rq/1(out) -> bus_creator/16  "PrkBrkMsgTxt_D_Rq"
  AccDis_B_ActlEpb/1(out) -> bus_creator/17  "AccDis_B_ActlEpb"
  CcDis_B_Cmd/1(out) -> bus_creator/18  "CcDis_B_Cmd"
  PrplDrgCtlActv_B_Actl/1(out) -> bus_creator/19  "PrplDrgCtlActv_B_Actl"
  AbsActv_B_Actl/1(out) -> bus_creator/20  "AbsActv_B_Actl"
  AccBrkDis_B_Actl/1(out) -> bus_creator/21  "AccBrkDis_B_Actl"
  AccBrkActv_B_Actl/1(out) -> bus_creator/22  "AccBrkActv_B_Actl"
  AccBrkDeny_B_Actl/1(out) -> bus_creator/23  "AccBrkDeny_B_Actl"
  VehLongOvrGnd_A_Est/1(out) -> bus_creator/24  "VehLongOvrGnd_A_Est"
  AccBrkWarm_B_Actl/1(out) -> bus_creator/25  "AccBrkWarm_B_Actl"
  AccBrkTotTqMn_B_Actl/1(out) -> bus_creator/26  "AccBrkTotTqMn_B_Actl"
  AccBrkPrchgActv_B_Actl/1(out) -> bus_creator/27  "AccBrkPrchgActv_B_Actl"
  CmbbDeny_B_ActlBrk/1(out) -> bus_creator/28  "CmbbDeny_B_ActlBrk"
  CmbbBrkPrchg_B_Actl/1(out) -> bus_creator/29  "CmbbBrkPrchg_B_Actl"
  CmbbBrkDecel_B_Actl/1(out) -> bus_creator/30  "CmbbBrkDecel_B_Actl"
  CmbbBaSensInc_B_Actl/1(out) -> bus_creator/31  "CmbbBaSensInc_B_Actl"
  CmbbBrkDis_B_Actl/1(out) -> bus_creator/32  "CmbbBrkDis_B_Actl"
  bus_selector/1 -> PrplWhlTot_Tq_RqMx/1(in)  "<PrplWhlTot_Tq_RqMx>"
  bus_selector/2 -> StabCtlBrkActv_B_Actl/1(in)  "<StabCtlBrkActv_B_Actl>"
  bus_selector/3 -> AccStopActv_B_ActlBrk/1(in)  "<AccStopActv_B_ActlBrk>"
  bus_selector/4 -> LscmbbBaSensInc_B_Actl/1(in)  "<LscmbbBaSensInc_B_Actl>"
  bus_selector/5 -> LscmbbBrkDecel_B_Actl/1(in)  "<LscmbbBrkDecel_B_Actl>"
  bus_selector/6 -> LscmbbBrkDis_B_Actl/1(in)  "<LscmbbBrkDis_B_Actl>"
  bus_selector/7 -> LscmbbDeny_B_ActlBrk/1(in)  "<LscmbbDeny_B_ActlBrk>"
  bus_selector/8 -> LscmbbMntr_B_Err/1(in)  "<LscmbbMntr_B_Err>"
  bus_selector/9 -> LscmbBrkPrchg_B_Actl/1(in)  "<LscmbBrkPrchg_B_Actl>"
  bus_selector/10 -> TracCtlPtActv_B_Actl/1(in)  "<TracCtlPtActv_B_Actl>"
  bus_selector/11 -> PrkBrkRedLamp_D_Rq/1(in)  "<PrkBrkRedLamp_D_Rq>"
  bus_selector/12 -> VehStop_D_Stat/1(in)  "<VehStop_D_Stat>"
  bus_selector/13 -> PrkBrkStatus/1(in)  "<PrkBrkStatus>"
  bus_selector/14 -> VehicleStationary/1(in)  "<VehicleStationary>"
  bus_selector/15 -> PrkBrkYwLamp_D_Rq/1(in)  "<PrkBrkYwLamp_D_Rq>"
  bus_selector/16 -> PrkBrkMsgTxt_D_Rq/1(in)  "<PrkBrkMsgTxt_D_Rq>"
  bus_selector/17 -> AccDis_B_ActlEpb/1(in)  "<AccDis_B_ActlEpb>"
  bus_selector/18 -> CcDis_B_Cmd/1(in)  "<CcDis_B_Cmd>"
  bus_selector/19 -> PrplDrgCtlActv_B_Actl/1(in)  "<PrplDrgCtlActv_B_Actl>"
  bus_selector/20 -> AbsActv_B_Actl/1(in)  "<AbsActv_B_Actl>"
  bus_selector/21 -> AccBrkDis_B_Actl/1(in)  "<AccBrkDis_B_Actl>"
  bus_selector/22 -> AccBrkActv_B_Actl/1(in)  "<AccBrkActv_B_Actl>"
  bus_selector/23 -> AccBrkDeny_B_Actl/1(in)  "<AccBrkDeny_B_Actl>"
  bus_selector/24 -> VehLongOvrGnd_A_Est/1(in)  "<VehLongOvrGnd_A_Est>"
  bus_selector/25 -> AccBrkWarm_B_Actl/1(in)  "<AccBrkWarm_B_Actl>"
  bus_selector/26 -> AccBrkTotTqMn_B_Actl/1(in)  "<AccBrkTotTqMn_B_Actl>"
  bus_selector/27 -> AccBrkPrchgActv_B_Actl/1(in)  "<AccBrkPrchgActv_B_Actl>"
  bus_selector/28 -> CmbbDeny_B_ActlBrk/1(in)  "<CmbbDeny_B_ActlBrk>"
  bus_selector/29 -> CmbbBrkPrchg_B_Actl/1(in)  "<CmbbBrkPrchg_B_Actl>"
  bus_selector/30 -> CmbbBrkDecel_B_Actl/1(in)  "<CmbbBrkDecel_B_Actl>"
  bus_selector/31 -> CmbbBaSensInc_B_Actl/1(in)  "<CmbbBaSensInc_B_Actl>"
  bus_selector/32 -> CmbbBrkDis_B_Actl/1(in)  "<CmbbBrkDis_B_Actl>"
  in/1 -> bus_selector/1

== system test_mdl_NI/CAN_Signal/ABS_ESC/DesiredTorqBrk_2_0x214 ==
  in : Inport
  PrplWhlRear_Tq_RqMn : Subsystem
  PrplWhlRear_Tq_RqMx : Subsystem
  PrplWhlTot_Tq_RqMn : Subsystem
  PrplWhlTqRqMn_No_Cnt : Subsystem
  PrplWhlTqRqMn_No_Cs : Subsystem
  RgenBrkDynoMde_B_Actl : Subsystem
  RgenTqFalt_B_Actl : Subsystem
  bus_creator : BusCreator  Inputs=7
  bus_selector : BusSelector  OutputSignals=PrplWhlTot_Tq_RqMn,PrplWhlRear_Tq_RqMx,PrplWhlRear_Tq_RqMn,PrplWhlTqRqMn_No_Cs,PrplWhlTqRqMn_No_Cnt,RgenTqFalt_B_Actl,RgenBrkDynoMde_B_Actl
  out_port : Outport
  wires:
  bus_creator/1 -> out_port/1  "DesiredTorqBrk_2_0x214"
  PrplWhlTot_Tq_RqMn/1(out) -> bus_creator/1  "PrplWhlTot_Tq_RqMn"
  PrplWhlRear_Tq_RqMx/1(out) -> bus_creator/2  "PrplWhlRear_Tq_RqMx"
  PrplWhlRear_Tq_RqMn/1(out) -> bus_creator/3  "PrplWhlRear_Tq_RqMn"
  PrplWhlTqRqMn_No_Cs/1(out) -> bus_creator/4  "PrplWhlTqRqMn_No_Cs"
  PrplWhlTqRqMn_No_Cnt/1(out) -> bus_creator/5  "PrplWhlTqRqMn_No_Cnt"
  RgenTqFalt_B_Actl/1(out) -> bus_creator/6  "RgenTqFalt_B_Actl"
  RgenBrkDynoMde_B_Actl/1(out) -> bus_creator/7  "RgenBrkDynoMde_B_Actl"
  bus_selector/1 -> PrplWhlTot_Tq_RqMn/1(in)  "<PrplWhlTot_Tq_RqMn>"
  bus_selector/2 -> PrplWhlRear_Tq_RqMx/1(in)  "<PrplWhlRear_Tq_RqMx>"
  bus_selector/3 -> PrplWhlRear_Tq_RqMn/1(in)  "<PrplWhlRear_Tq_RqMn>"
  bus_selector/4 -> PrplWhlTqRqMn_No_Cs/1(in)  "<PrplWhlTqRqMn_No_Cs>"
  bus_selector/5 -> PrplWhlTqRqMn_No_Cnt/1(in)  "<PrplWhlTqRqMn_No_Cnt>"
  bus_selector/6 -> RgenTqFalt_B_Actl/1(in)  "<RgenTqFalt_B_Actl>"
  bus_selector/7 -> RgenBrkDynoMde_B_Actl/1(in)  "<RgenBrkDynoMde_B_Actl>"
  in/1 -> bus_selector/1

== system test_mdl_NI/CAN_Signal/ABS_ESC/Global_PATS_SubTarget_0x49 ==
  in : Inport
  bus_creator : BusCreator  Inputs=2
  bus_selector : BusSelector  OutputSignals=immoSubTarget1Cmd_T1,immoSubTarget1Data_T1
  immoSubTarget1Cmd_T1 : Subsystem
  immoSubTarget1Data_T1 : Subsystem
  out_port : Outport
  wires:
  bus_creator/1 -> out_port/1  "Global_PATS_SubTarget_0x49"
  immoSubTarget1Cmd_T1/1(out) -> bus_creator/1  "immoSubTarget1Cmd_T1"
  immoSubTarget1Data_T1/1(out) -> bus_creator/2  "immoSubTarget1Data_T1"
  bus_selector/1 -> immoSubTarget1Cmd_T1/1(in)  "<immoSubTarget1Cmd_T1>"
  bus_selector/2 -> immoSubTarget1Data_T1/1(in)  "<immoSubTarget1Data_T1>"
  in/1 -> bus_selector/1

== system test_mdl_NI/CAN_Signal/ABS_ESC/SelectDriveModeData2_0x44E ==
  in : Inport
  SelDrvMdePos01_D_Stat : Subsystem
  SelDrvMdePos02_D_Stat : Subsystem
  SelDrvMdePos03_D_Stat : Subsystem
  SelDrvMdePos04_D_Stat : Subsystem
  SelDrvMdePos05_D_Stat : Subsystem
  SelDrvMdePos06_D_Stat : Subsystem
  SelDrvMdePos07_D_Stat : Subsystem
  SelDrvMdePos08_D_Stat : Subsystem
  SelDrvMdePos09_D_Stat : Subsystem
  SelDrvMdePos10_D_Stat : Subsystem
  SelDrvMdePos11_D_Stat : Subsystem
  SelDrvMdePos12_D_Stat : Subsystem
  bus_creator : BusCreator  Inputs=12
  bus_selector : BusSelector  OutputSignals=SelDrvMdePos01_D_Stat,SelDrvMdePos02_D_Stat,SelDrvMdePos03_D_Stat,SelDrvMdePos04_D_Stat,SelDrvMdePos05_D_Stat,SelDrvMdePos06_D_Stat,SelDrvMdePos07_D_Stat,SelDrvMdePos12_D_Stat,SelDrvMdePos11_D_Stat,SelDrvMdePos10_D_Stat,SelDrvMdePos09_D_Stat,SelDrvMdePos08_D_Stat
  out_port : Outport
  wires:
  bus_creator/1 -> out_port/1  "SelectDriveModeData2_0x44E"
  SelDrvMdePos01_D_Stat/1(out) -> bus_creator/1  "SelDrvMdePos01_D_Stat"
  SelDrvMdePos02_D_Stat/1(out) -> bus_creator/2  "SelDrvMdePos02_D_Stat"
  SelDrvMdePos03_D_Stat/1(out) -> bus_creator/3  "SelDrvMdePos03_D_Stat"
  SelDrvMdePos04_D_Stat/1(out) -> bus_creator/4  "SelDrvMdePos04_D_Stat"
  SelDrvMdePos05_D_Stat/1(out) -> bus_creator/5  "SelDrvMdePos05_D_Stat"
  SelDrvMdePos06_D_Stat/1(out) -> bus_creator/6  "SelDrvMdePos06_D_Stat"
  SelDrvMdePos07_D_Stat/1(out) -> bus_creator/7  "SelDrvMdePos07_D_Stat"
  SelDrvMdePos12_D_Stat/1(out) -> bus_creator/8  "SelDrvMdePos12_D_Stat"
  SelDrvMdePos11_D_Stat/1(out) -> bus_creator/9  "SelDrvMdePos11_D_Stat"
  SelDrvMdePos10_D_Stat/1(out) -> bus_creator/10  "SelDrvMdePos10_D_Stat"
  SelDrvMdePos09_D_Stat/1(out) -> bus_creator/11  "SelDrvMdePos09_D_Stat"
  SelDrvMdePos08_D_Stat/1(out) -> bus_creator/12  "SelDrvMdePos08_D_Stat"
  bus_selector/1 -> SelDrvMdePos01_D_Stat/1(in)  "<SelDrvMdePos01_D_Stat>"
  bus_selector/2 -> SelDrvMdePos02_D_Stat/1(in)  "<SelDrvMdePos02_D_Stat>"
  bus_selector/3 -> SelDrvMdePos03_D_Stat/1(in)  "<SelDrvMdePos03_D_Stat>"
  bus_selector/4 -> SelDrvMdePos04_D_Stat/1(in)  "<SelDrvMdePos04_D_Stat>"
  bus_selector/5 -> SelDrvMdePos05_D_Stat/1(in)  "<SelDrvMdePos05_D_Stat>"
  bus_selector/6 -> SelDrvMdePos06_D_Stat/1(in)  "<SelDrvMdePos06_D_Stat>"
  bus_selector/7 -> SelDrvMdePos07_D_Stat/1(in)  "<SelDrvMdePos07_D_Stat>"
  bus_selector/8 -> SelDrvMdePos12_D_Stat/1(in)  "<SelDrvMdePos12_D_Stat>"
  bus_selector/9 -> SelDrvMdePos11_D_Stat/1(in)  "<SelDrvMdePos11_D_Stat>"
  bus_selector/10 -> SelDrvMdePos10_D_Stat/1(in)  "<SelDrvMdePos10_D_Stat>"
  bus_selector/11 -> SelDrvMdePos09_D_Stat/1(in)  "<SelDrvMdePos09_D_Stat>"
  bus_selector/12 -> SelDrvMdePos08_D_Stat/1(in)  "<SelDrvMdePos08_D_Stat>"
  in/1 -> bus_selector/1

== system test_mdl_NI/CAN_Signal/ABS_ESC/SelectDriveModeData_0x420 ==
  in : Inport
  ActvDrvMde_D2_Stat : Subsystem
  AwdMde_D_RqBrk : Subsystem
  SelDrvMdeMsgTxt_D_Rq : Subsystem
  SelDrvMdePos01_B_Avail : Subsystem
  SelDrvMdePos02_B_Avail : Subsystem
  SelDrvMdePos03_B_Avail : Subsystem
  SelDrvMdePos04_B_Avail : Subsystem
  SelDrvMdePos05_B_Avail : Subsystem
  SelDrvMdePos06_B_Avail : Subsystem
  SelDrvMdePos07_B_Avail : Subsystem
  SelDrvMdePos08_B_Avail : Subsystem
  SelDrvMdePos09_B_Avail : Subsystem
  SelDrvMdePos10_B_Avail : Subsystem
  SelDrvMdePos11_B_Avail : Subsystem
  SelDrvMdePos12_B_Avail : Subsystem
  SelDrvMdePt_D_Rq : Subsystem
  SelDrvMde_D2_Rq : Subsystem
  SelDrvMde_D_Stat : Subsystem
  bus_creator : BusCreator  Inputs=18
  bus_selector : BusSelector  OutputSignals=SelDrvMdeMsgTxt_D_Rq,SelDrvMdePt_D_Rq,SelDrvMde_D_Stat,SelDrvMdePos01_B_Avail,AwdMde_D_RqBrk,SelDrvMdePos02_B_Avail,SelDrvMdePos03_B_Avail,SelDrvMdePos04_B_Avail,SelDrvMdePos05_B_Avail,SelDrvMdePos06_B_Avail,SelDrvMdePos07_B_Avail,SelDrvMdePos08_B_Avail,SelDrvMdePos09_B_Avail,SelDrvMdePos10_B_Avail,SelDrvMdePos11_B_Avail,SelDrvMdePos12_B_Avail,ActvDrvMde_D2_Stat,SelDrvMde_D2_Rq
  out_port : Outport
  wires:
  bus_creator/1 -> out_port/1  "SelectDriveModeData_0x420"
  SelDrvMdeMsgTxt_D_Rq/1(out) -> bus_creator/1  "SelDrvMdeMsgTxt_D_Rq"
  SelDrvMdePt_D_Rq/1(out) -> bus_creator/2  "SelDrvMdePt_D_Rq"
  SelDrvMde_D_Stat/1(out) -> bus_creator/3  "SelDrvMde_D_Stat"
  SelDrvMdePos01_B_Avail/1(out) -> bus_creator/4  "SelDrvMdePos01_B_Avail"
  AwdMde_D_RqBrk/1(out) -> bus_creator/5  "AwdMde_D_RqBrk"
  SelDrvMdePos02_B_Avail/1(out) -> bus_creator/6  "SelDrvMdePos02_B_Avail"
  SelDrvMdePos03_B_Avail/1(out) -> bus_creator/7  "SelDrvMdePos03_B_Avail"
  SelDrvMdePos04_B_Avail/1(out) -> bus_creator/8  "SelDrvMdePos04_B_Avail"
  SelDrvMdePos05_B_Avail/1(out) -> bus_creator/9  "SelDrvMdePos05_B_Avail"
  SelDrvMdePos06_B_Avail/1(out) -> bus_creator/10  "SelDrvMdePos06_B_Avail"
  SelDrvMdePos07_B_Avail/1(out) -> bus_creator/11  "SelDrvMdePos07_B_Avail"
  SelDrvMdePos08_B_Avail/1(out) -> bus_creator/12  "SelDrvMdePos08_B_Avail"
  SelDrvMdePos09_B_Avail/1(out) -> bus_creator/13  "SelDrvMdePos09_B_Avail"
  SelDrvMdePos10_B_Avail/1(out) -> bus_creator/14  "SelDrvMdePos10_B_Avail"
  SelDrvMdePos11_B_Avail/1(out) -> bus_creator/15  "SelDrvMdePos11_B_Avail"
  SelDrvMdePos12_B_Avail/1(out) -> bus_creator/16  "SelDrvMdePos12_B_Avail"
  ActvDrvMde_D2_Stat/1(out) -> bus_creator/17  "ActvDrvMde_D2_Stat"
  SelDrvMde_D2_Rq/1(out) -> bus_creator/18  "SelDrvMde_D2_Rq"
  bus_selector/1 -> SelDrvMdeMsgTxt_D_Rq/1(in)  "<SelDrvMdeMsgTxt_D_Rq>"
  bus_selector/2 -> SelDrvMdePt_D_Rq/1(in)  "<SelDrvMdePt_D_Rq>"
  bus_selector/3 -> SelDrvMde_D_Stat/1(in)  "<SelDrvMde_D_Stat>"
  bus_selector/4 -> SelDrvMdePos01_B_Avail/1(in)  "<SelDrvMdePos01_B_Avail>"
  bus_selector/5 -> AwdMde_D_RqBrk/1(in)  "<AwdMde_D_RqBrk>"
  bus_selector/6 -> SelDrvMdePos02_B_Avail/1(in)  "<SelDrvMdePos02_B_Avail>"
  bus_selector/7 -> SelDrvMdePos03_B_Avail/1(in)  "<SelDrvMdePos03_B_Avail>"
  bus_selector/8 -> SelDrvMdePos04_B_Avail/1(in)  "<SelDrvMdePos04_B_Avail>"
  bus_selector/9 -> SelDrvMdePos05_B_Avail/1(in)  "<SelDrvMdePos05_B_Avail>"
  bus_selector/10 -> SelDrvMdePos06_B_Avail/1(in)  "<SelDrvMdePos06_B_Avail>"
  bus_selector/11 -> SelDrvMdePos07_B_Avail/1(in)  "<SelDrvMdePos07_B_Avail>"
  bus_selector/12 -> SelDrvMdePos08_B_Avail/1(in)  "<SelDrvMdePos08_B_Avail>"
  bus_selector/13 -> SelDrvMdePos09_B_Avail/1(in)  "<SelDrvMdePos09_B_Avail>"
  bus_selector/14 -> SelDrvMdePos10_B_Avail/1(in)  "<SelDrvMdePos10_B_Avail>"
  bus_selector/15 -> SelDrvMdePos11_B_Avail/1(in)  "<SelDrvMdePos11_B_Avail>"
  bus_selector/16 -> SelDrvMdePos12_B_Avail/1(in)  "<SelDrvMdePos12_B_Avail>"
  bus_selector/17 -> ActvDrvMde_D2_Stat/1(in)  "<ActvDrvMde_D2_Stat>"
  bus_selector/18 -> SelDrvMde_D2_Rq/1(in)  "<SelDrvMde_D2_Rq>"
  in/1 -> bus_selector/1

== system test_mdl_NI/CAN_Signal/ABS_ESC/SteeringPinion_Data2_0x7F ==
  in : Inport
  AwdLatDelta_B_Rq : Subsystem
  AwdLatDelta_Tq_Rq : Subsystem
  bus_creator : BusCreator  Inputs=2
  bus_selector : BusSelector  OutputSignals=AwdLatDelta_B_Rq,AwdLatDelta_Tq_Rq
  out_port : Outport
  wires:
  bus_creator/1 -> out_port/1  "SteeringPinion_Data2_0x7F"
  AwdLatDelta_B_Rq/1(out) -> bus_creator/1  "AwdLatDelta_B_Rq"
  AwdLatDelta_Tq_Rq/1(out) -> bus_creator/2  "AwdLatDelta_Tq_Rq"
  bus_selector/1 -> AwdLatDelta_B_Rq/1(in)  "<AwdLatDelta_B_Rq>"
  bus_selector/2 -> AwdLatDelta_Tq_Rq/1(in)  "<AwdLatDelta_Tq_Rq>"
  in/1 -> bus_selector/1
